simulink model "dc_motor"  (R2020b)
settings: Solver=VariableStepAuto  StartTime=0.0  StopTime=20  RelTol=1e-3
settings Model: Creator=kjartan  LastModifiedBy=kjartan

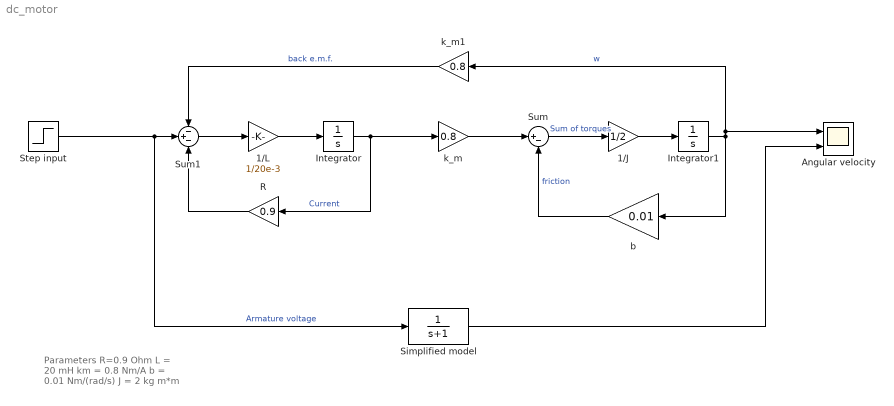
== system dc_motor ==
  note: Parameters
      |
      | R=0.9 Ohm
      | L = 20 mH
      | km = 0.8 Nm/A
      | b = 0.01 Nm/(rad/s)
      | J = 2 kg m*m
  1/J : Gain  Gain=1/2
  1/L : Gain  Gain=1/20e-3
  Angular velocity : Scope  NumInputPorts=2
  Integrator : Integrator
  Integrator1 : Integrator
  R : Gain  Gain=0.9
  Simplified model : TransferFcn  Denominator=[1 1]
  Step input : Step  After=100  SampleTime=0
  Sum : Sum  Inputs=|+-
  Sum1 : Sum  Inputs=-+-
  b : Gain  Gain=0.01
  k_m : Gain  Gain=0.8
  k_m1 : Gain  Gain=0.8
  wires:
  1/J/1 -> Integrator1/1
  Integrator1/1 -> k_m1/1, Angular velocity/1, b/1  "w"
  Sum/1 -> 1/J/1  "Sum of torques"
  b/1 -> Sum/2  "friction"
  k_m/1 -> Sum/1
  Integrator/1 -> R/1, k_m/1  "Current"
  1/L/1 -> Integrator/1
  R/1 -> Sum1/3
  Sum1/1 -> 1/L/1
  k_m1/1 -> Sum1/1  "back e.m.f."
  Step input/1 -> Simplified model/1, Sum1/2  "Armature voltage"
  Simplified model/1 -> Angular velocity/2
